simulink model "Kalman_MPPT"  (R2018a)
settings: Solver=ode23tb  StartTime=0.0  StopTime=3  RelTol=1e-3
undefined symbols (not defined in the file): sigbuilder_block
libraries: powerlib x10, re_lib x1, powerlib_meascontrol x1
settings Model: Creator=msidd  LastModifiedBy=msidd

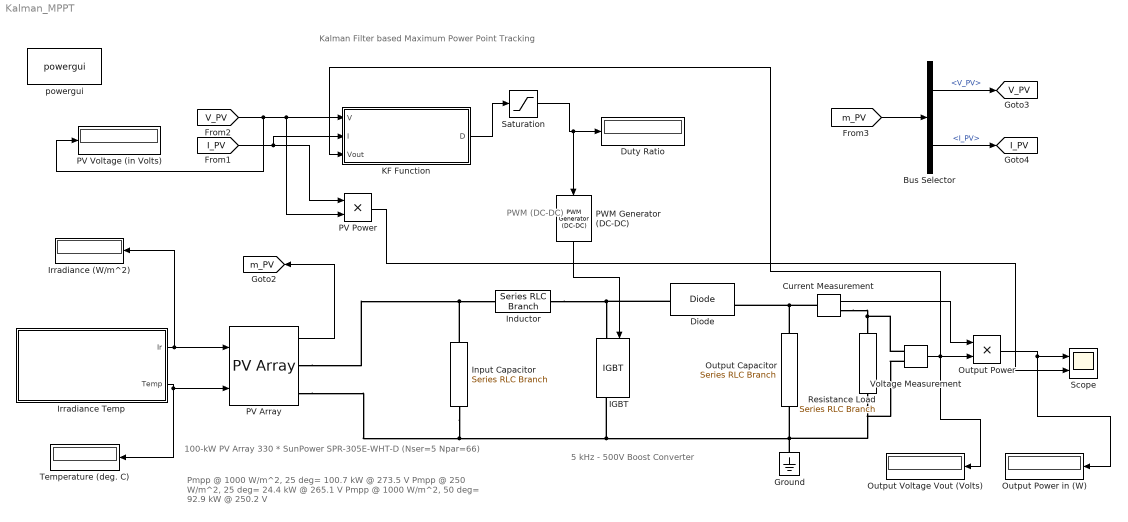
== system Kalman_MPPT ==
  note: PWM
      | (DC-DC)
  note: Kalman Filter based Maximum Power Point Tracking
  note: 100-kW  PV Array
      | 330 * SunPower SPR-305E-WHT-D  (Nser=5 Npar=66)
  note: Pmpp @ 1000 W/m^2, 25 deg= 100.7 kW @ 273.5 V
      | Pmpp @  250 W/m^2, 25 deg= 24.4  kW @ 265.1 V
      | Pmpp @ 1000 W/m^2, 50 deg= 92.9  kW @ 250.2 V
  note: 5 kHz - 500V
      | Boost Converter
  " Resistance Load      " : powerlib/Elements/Series RLC Branch  LConnTagsString=__new0  RConnTagsString=__new0  BranchType=R  Resistance=2.5  Inductance=1e-3  SetiL0=off  InitialCurrent=0  Capacitance=1e-6  Setx0=off  InitialVoltage=0  Measurements=None
  " Output Capacitor   " : powerlib/Elements/Series RLC Branch  LConnTagsString=__new0  RConnTagsString=__new0  BranchType=C  Resistance=1  Inductance=1e-3  SetiL0=off  InitialCurrent=0  Capacitance=12000e-6  Setx0=off  InitialVoltage=0  Measurements=None
  Bus Selector : BusSelector  OutputSignals=V_PV,I_PV
  Current Measurement : powerlib/Measurements/Current Measurement  PhasorSimulation=off  OutputType=Complex  PSBequivalent=0
  "Diode " : powerlib/Power Electronics/Diode  Ron=0.001  Lon=0  Vf=0.8  IC=0  UseSnubber=0  Rs=500  Cs=250e-9  Measurements=on
  Duty Ratio : Display
      settings: Format=bank  Decimation=1000
  Ground : powerlib/Elements/Ground  LConnTagsString=a
  "IGBT  " : powerlib/Power Electronics/IGBT  Ron=0.001  Lon=0  Vf=1  Tf=1e-6  Tt=2e-6  IC=0  Rs=1e5  Cs=inf  Measurements=on
  "Inductor " : powerlib/Elements/Series RLC Branch  LConnTagsString=__new0  RConnTagsString=__new0  BranchType=L  Resistance=0.005  Inductance=5e-3  SetiL0=off  InitialCurrent=0  Capacitance=1e-6  Setx0=off  InitialVoltage=0  Measurements=None
  "Input Capacitor " : powerlib/Elements/Series RLC Branch  LConnTagsString=__new0  RConnTagsString=__new0  BranchType=C  Resistance=1  Inductance=1e-3  SetiL0=off  InitialCurrent=0  Capacitance=100e-6  Setx0=off  InitialVoltage=0  Measurements=None
  Irradiance (W/m^2) : Display
      settings: Format=bank  Decimation=1000
  Irradiance Temp : Subsystem  Tag=STV Subsys  LoadFcn=sigbuilder_block('load');  StartFcn=sigbuilder_block('start');  StopFcn=sigbuilder_block('stop');  ClipboardFcn=sigbuilder_block('clipboard');  mask(Sigbuilder block){tuvar=[0:10]}
      mask help: Sigbuilder GUI
      mask init:
      | if ~strcmp(get_param(bdroot(gcbh),'SimulationStatus'),'stopped') tuvar = sigbuilder_block('maskInit'); end
      settings: CopyFcn=sigbuilder_block('copy');  DeleteFcn=sigbuilder_block('delete');  ModelCloseFcn=sigbuilder_block('modelClose');  PreSaveFcn=sigbuilder_block('preSave');  PauseFcn=sigbuilder_block('pause')  ContinueFcn=sigbuilder_block('continue')  NameChangeFcn=sigbuilder_block('namechange');  OpenFcn=sigbuilder_block('open',[220.5 133.5 543.5 346.5 ]);  CloseFcn=sigbuilder_block('close');
      mask Display: plot(0, 0, 100, 100,[2, 2, 32, 32, 2], [68, 8, 8, 68, 68],[32, 2], [38, 38], [32, 19, 2],[53, 60, 44], [32, 17, 17, 2],[16, 16, 31, 31]);txt = getActiveGroup(gcbh);text(2, 100, txt,'verticalAlignment', 'top');
  KF Function : MATLAB Function  TreatAsAtomicUnit=on
  Output Power : Product
  Output Power in (W) : Display
      settings: Format=bank  Decimation=1000
  Output Voltage Vout (Volts) : Display
      settings: Format=bank  Decimation=1000
  PV Array : re_lib/Solar/PV Array  Npar=66  Nser=5  PlotType=array @ 1000 W/m2 & specified temperatures  S_vec="[ 1000  500  100 ]"  Temp_C_vec="[ 45 25  ]"  ModuleName=SunPower SPR-305E-WHT-D  PlotWhenSelected=off  Pm=305.226  Ncell=96  Voc=64.2  Isc=5.96  Vm=54.7  Im=5.58  beta_Voc_pc=-0.27269  alpha_Isc_pc=0.061745  beta_Voc=-0.17507  alpha_Isc=0.00368  IL=6.0092  I0=6.3014e-12  nI=0.94504  Rsh=269.5934  Rs=0.37152  BAL=on  Tc=1e-6  Tfilter=5e-5
  PV Power : Product
  PV Voltage (in Volts) : Display
  PWM Generator (DC-DC) : powerlib_meascontrol/Pulse & Signal Generators/PWM Generator (DC-DC)  Fsw=5000  Ts=1e-6
  "Saturation " : Saturate  UpperLimit=1  LowerLimit=0
  Scope : Scope  NumInputPorts=2
  Temperature (deg. C) : Display
      settings: Format=bank  Decimation=1000
  Voltage Measurement : powerlib/Measurements/Voltage Measurement  PhasorSimulation=off  OutputType=Complex  PSBequivalent=0
  powergui : powerlib/powergui  Priority=1  SimulationMode=Discrete  SampleTime=1e-6  frequency=60  Iterations=50  frequencyindice=0  Pbase=100e6  ErrMax=1e-4  UnitsV=kV  UnitsW=MW  buscounter=0  FunctionMessages=off  echomessages=off  EnableUseOfTLC=off  CurrentSourceSwitches=off  DisableSnubberDevices=off  DisableRonSwitches=off  DisableVfSwitches=off  DisplayEquations=off  SolverType=Tustin/Backward Euler (TBE)  Interpol=off  ExternalGateDelay=off  methode=off  Ts=100  x0status=blocks  SPID=on  SwTol=0  HookPort=off  RestoreLinks=warning  ResistiveCurrentMeasurement=off  Frange=[0:2:500]  Ylog=off  Xlog=on  ShowGrid=off  save=off  variable=ZData  structure=0  ZoomFFT=off  StartTime=0.0  cycles=1  DisplayStyle=1  fundamental=60  FreqAxis=off  MaxFrequency=1000  frequencyindicesteady=1  RmsSteady=1  display=off
  tag scope: I_PV=global, V_PV=global, m_PV=global
  wires:
  Voltage Measurement/1 -> KF Function/3(Vout), Output Voltage Vout (Volts)/1, Output Power/2
  Current Measurement/1 -> Output Power/1
  Output Power/1 -> Output Power in (W)/1, Scope/1
  [V_PV] -> PV Voltage (in Volts)/1, PV Power/2, KF Function/1(V)
  [I_PV] -> PV Power/1, KF Function/2(I)
  Irradiance Temp/2(Temp) -> Temperature (deg. C)/1, PV Array/2
  Irradiance Temp/1(Ir) -> Irradiance (W/m^2)/1, PV Array/1
  PV Array/1 -> [m_PV]
  Bus Selector/1 -> [V_PV]  "<V_PV>"
  [m_PV] -> Bus Selector/1
  Bus Selector/2 -> [I_PV]  "<I_PV>"
  "Saturation "/1 -> Duty Ratio/1, PWM Generator (DC-DC)/1
  KF Function/1(D) -> "Saturation "/1
  PWM Generator (DC-DC)/1 -> "IGBT  "/1
  PV Power/1 -> Scope/2
  connections:
  PV Array/RConn1 -- "Input Capacitor "/LConn1 -- "Inductor "/LConn1
  "Inductor "/RConn1 -- "Diode "/LConn1 -- "IGBT  "/LConn1
  PV Array/RConn2 -- "Input Capacitor "/RConn1 -- "IGBT  "/RConn1 -- Voltage Measurement/LConn2 -- " Resistance Load      "/RConn1 -- Ground/LConn1 -- " Output Capacitor   "/RConn1
  Current Measurement/LConn1 -- " Output Capacitor   "/LConn1 -- "Diode "/RConn1
  Current Measurement/RConn1 -- Voltage Measurement/LConn1 -- " Resistance Load      "/LConn1

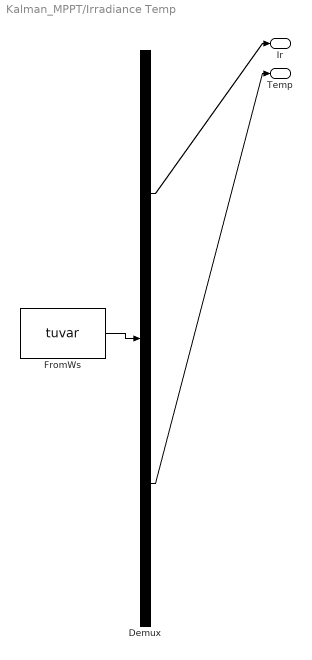
== system Kalman_MPPT/Irradiance Temp ==
  Demux : Demux  Tag=STV Demux  Outputs=2
  FromWs : FromWorkspace  Tag=STV FromWs  VariableName=tuvar  SampleTime=0
      SigBuilderData=|
      | common.afterFinalStr = 'Extrapolate'
      | common.sampleTime = '0'
      | dataSet(1).timeRange = [0 2]
      | dataSet(1).name = 'Constant Irradiance'
      | dataSet(2).timeRange = [0 2]
      | dataSet(2).name = 'Step Irradiance'
      | dataSet(3).timeRange = [0 3]
      | dataSet(3).name = 'Ramp-up/down Irradiance'
      | sbobj.Groups(1).Name = 'Constant Irradiance'
      | sbobj.Groups(1).Signals(1).Name = 'Ir'
      | sbobj.Groups(1).Signals(1).XData = [0 2]
      | sbobj.Groups(1).Signals(1).YData = [1000 1000]
      | sbobj.Groups(1).Signals(2).Name = 'Temp'
      | sbobj.Groups(1).Signals(2).XData = [0 1 2]
      | sbobj.Groups(1).Signals(2).YData = [25 25 25]
      | sbobj.Groups(1).TimeRange = [0 2]
      | sbobj.Groups(2).Name = 'Step Irradiance'
      | sbobj.Groups(2).Signals(1).Name = 'Ir'
      | sbobj.Groups(2).Signals(1).XData = [0 0.252 2]
      | sbobj.Groups(2).Signals(1).YData = [1000 1000 1000]
      | sbobj.Groups(2).Signals(2).Name = 'Temp'
      | sbobj.Groups(2).Signals(2).XData = [0 1 2]
      | sbobj.Groups(2).Signals(2).YData = [25 25 25]
      | sbobj.Groups(2).TimeRange = [0 2]
      | sbobj.Groups(3).Name = 'Ramp-up/down Irradiance'
      | sbobj.Groups(3).Signals(1).Name = 'Ir'
      | sbobj.Groups(3).Signals(1).XData = [0 0.6 1.1 1.2 1.7 1.7 3]
      | sbobj.Groups(3).Signals(1).YData = [1000 1000 250 250 1000 1000 1000]
      | sbobj.Groups(3).Signals(2).Name = 'Temp'
      | sbobj.Groups(3).Signals(2).XData = [0 2 2.1 3]
      | sbobj.Groups(3).Signals(2).YData = [25 25 50 50]
      | sbobj.Groups(3).TimeRange = [0 3]
  Ir : Outport  Tag=STV Outport
  Temp : Outport  Tag=STV Outport  Port=2
  wires:
  Demux/1 -> Ir/1
  FromWs/1 -> Demux/1
  Demux/2 -> Temp/1

== matlab function Kalman_MPPT/KF Function ==
  data: V input; D output; I input; Vout input
function D = KalmanFilter(V, I, Vout)

% PARAMETERS DEFINATION
A = 1; %Matrix A
step = 5; %step size
B = step; %Matrix B
C = 1; %Matrix C
Vmpp = 273.5; %Maximum power point voltage (in volts)
Impp = 368.28; %Maximum power point current (in Amp)
Q = 50; 
R = 50;

% KF PARAMETERS INTIALISATION
%STEP-I
persistent v_k
if isempty(v_k)
    v_k = Vmpp;
end
persistent power_k
if isempty(power_k)
    power_k = Vmpp*Impp;
end
persistent v_k_prev
if isempty(v_k_prev)
    v_k_prev = 0;
end
persistent power_k_prev
if isempty(power_k_prev)
    power_k_prev = 0;
end
persistent h_k
if isempty(h_k)
    h_k = 1;
end

pv_slope = (power_k - power_k_prev)/(v_k - v_k_prev);

%KF IMPLEMENTATION
% STAGE - PREDICTION
%STEP-II: Project the state ahead
v_neg = v_k + step*pv_slope;

%STEP-III: Project the error covariance ahead
h_neg = h_k + Q;

% STAGE - UPDATION
% STEP-IV: Compute the kalman gain
K_ = (h_neg)/(h_neg + R);

% STEP-V: Update estimate with measurement Vout
v = v_neg + K_*(V - v_neg);

% STEP-VI: Update the error covariance
h = (1-K_)*h_neg;

% STEP-VII: Saving for next stage
h_k = h;
v_k_prev = v_k;
power_k_prev = power_k;
v_k = V;
power_k = V*I;

% OUTPUT DUTY CYCLE
D = 1 - (v/Vout);
end
